simulink model "Sim3_Cart_OA"  (R2021b)
settings: Solver=VariableStepAuto  StartTime=0.0  StopTime=Inf  RelTol=1e-3
InitFcn:
  | run('settingParams.m')
undefined symbols (not defined in the file or in its folder): dt, Init_Direction, StartPoint, TurnPoint, Twist
libraries: robotlib x5, instrumentseriallib x4, simulink x1, realtime_pacer_lib x1
settings Model: Creator=shdet  LastModifiedBy=Hibik
settings SolverCC: AlgebraicLoopSolver=TrustRegion
settings DataIOCC: SaveOutput=off  SignalLogging=off  DSMLogging=off  SaveTime=off  ReturnWorkspaceOutputs=off
settings DebuggingCC: PregeneratedLibrarySubsystemCodeDiagnostic=none  SFMachineParentedDataDiag=warning  ArithmeticOperatorsInVariantConditions=warning
settings SFSimCC: SimUseLocalCustomCode=off  CustomCodeUndefinedFunction=UseInterfaceOnly
settings RTWCC: RTWUseLocalCustomCode=off

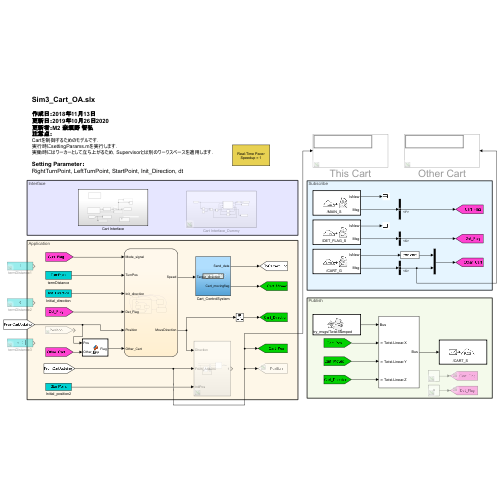
[thumbnail: Simulink's stored preview of the top-level diagram]
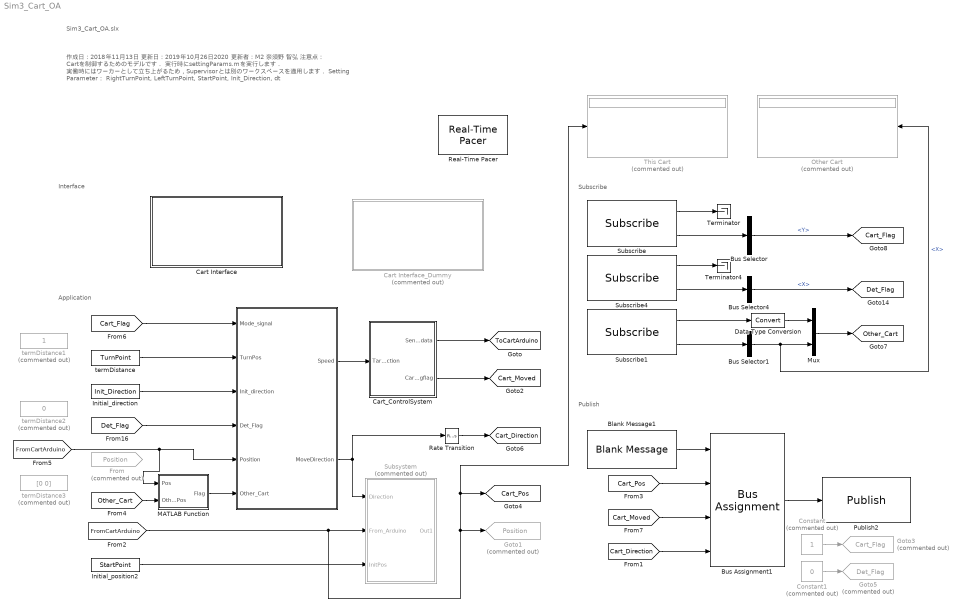
== system Sim3_Cart_OA ==
  note: 作成日：2018年11月13日
      | 更新日：2019年10月26日2020
      | 更新者：M2 奈須野 智弘
      | 注意点：
      | Cartを制御するためのモデルです．
      | 実行時にsettingParams.mを実行します．
      | 実働時にはワーカーとして立ち上がるため，Supervisorとは別のワークスペースを適用します．
      |
      | Setting Parameter：
      | RightTurnPoint, LeftTurnPoint, StartPoint, Init_Direction, dt
  note: Sim3_Cart_OA.slx
  note: Subscribe
  note: Publish
  note: Application
  note: Interface
  " " : Stateflow chart  TreatAsAtomicUnit=on
  Blank Message1 : robotlib/Blank Message  messageClass=Message  entityType=geometry_msgs/TwistStamped  messageType=geometry_msgs/TwistStamped  SampleTime=inf  legacyBusStruct=off
  Bus Assignment1 : BusAssignment  AssignedSignals=Twist.Linear.X,Twist.Linear.Y,Twist.Linear.Z
  Bus Selector : BusSelector  OutputSignals=Twist.Linear.Y
  Bus Selector1 : BusSelector  OutputSignals=Twist.Linear.X
  Bus Selector4 : BusSelector  OutputSignals=Twist.Linear.X
  Cart Interface : Subsystem
  Cart Interface_Dummy : Subsystem  Commented=on
  Cart_ControlSystem : Subsystem
  Constant : Constant  Commented=on  SampleTime=dt
  Constant1 : Constant  Commented=on  Value=0  SampleTime=dt
  Data Type Conversion : DataTypeConversion
  From : From  Commented=on  GotoTag=Position  TagVisibility=global
  Goto1 : Goto  Commented=on  GotoTag=Position  TagVisibility=global
  Goto3 : Goto  Commented=on  GotoTag=Cart_Flag  TagVisibility=global
  Goto5 : Goto  Commented=on  GotoTag=Det_Flag  TagVisibility=global
  Initial_direction : Constant  Value=Init_Direction  SampleTime=dt
  Initial_position2 : Constant  Value=StartPoint  SampleTime=dt
  MATLAB Function : MATLAB Function  TreatAsAtomicUnit=on
  Mux : Mux  Inputs=2
  Other Cart : Display  Commented=on
  Publish2 : robotlib/Publish  topicSource=Specify your own  topic=/CART_S  messageType=geometry_msgs/TwistStamped  legacyBusStruct=off  messageQueueLength=1
  Rate Transition : RateTransition
  Real-Time Pacer : realtime_pacer_lib/Real-Time Pacer  simTimePerRealTime=1
      settings: SourceProductName=Real-Time Pacer
  Subscribe : robotlib/Subscribe  topicSource=Specify your own  topic=/MAIN_S  messageType=geometry_msgs/TwistStamped  SampleTime=-1  legacyBusStruct=off  messageQueueLength=1
  Subscribe1 : robotlib/Subscribe  topicSource=Specify your own  topic=/CART_G  messageType=geometry_msgs/TwistStamped  SampleTime=-1  legacyBusStruct=off  messageQueueLength=1
  Subscribe4 : robotlib/Subscribe  topicSource=Specify your own  topic=/DET_FLAG_S  messageType=geometry_msgs/TwistStamped  SampleTime=-1  legacyBusStruct=off  messageQueueLength=1
  Subsystem : Subsystem  Commented=on
  Terminator : Terminator
  Terminator4 : Terminator
  This Cart : Display  Commented=on
  termDistance : Constant  Value=TurnPoint  SampleTime=dt
  termDistance1 : Constant  Commented=on  SampleTime=dt
  termDistance2 : Constant  Commented=on  Value=0  SampleTime=dt
  termDistance3 : Constant  Commented=on  Value=[0 0]  SampleTime=dt
  tag scope: Cart_Direction=global, Cart_Flag=global, Cart_Moved=global, Cart_Pos=global, Det_Flag=global, Other_Cart=global, ToCartArduino=global
  wires:
  Subscribe4/2 -> Bus Selector4/1
  Subscribe4/1 -> Terminator4/1
  [Cart_Pos] -> Bus Assignment1/2
  Bus Assignment1/1 -> Publish2/1
  Bus Selector4/1 -> [Det_Flag]  "<X>"
  Subscribe/1 -> Terminator/1
  [Cart_Moved] -> Bus Assignment1/3
  Blank Message1/1 -> Bus Assignment1/1
  Subscribe/2 -> Bus Selector/1
  Bus Selector/1 -> [Cart_Flag]  "<Y>"
  Cart_ControlSystem/2(Cart_movingflag) -> [Cart_Moved]
  Cart_ControlSystem/1(Send_data) -> [ToCartArduino]
  termDistance/1 -> " "/2(TurnPos)
  " "/1(Speed) -> Cart_ControlSystem/1(Target_direction)
  Initial_direction/1 -> " "/3(Init_direction)
  " "/2(MoveDirection) -> Rate Transition/1, Subsystem/1(Direction)
  [FromCartArduino] -> This Cart/1, [Cart_Pos], Goto1/1, Subsystem/2(From_Arduino)
  [Cart_Direction] -> Bus Assignment1/4
  Constant1/1 -> Goto5/1
  Constant/1 -> Goto3/1
  Bus Selector1/1 -> Other Cart/1, Mux/2  "<X>"
  Subscribe1/2 -> Bus Selector1/1
  Subscribe1/1 -> Data Type Conversion/1
  Mux/1 -> [Other_Cart]
  Data Type Conversion/1 -> Mux/1
  Rate Transition/1 -> [Cart_Direction]
  MATLAB Function/1(Flag) -> " "/6(Other_Cart)
  Initial_position2/1 -> Subsystem/3(InitPos)
  [FromCartArduino] -> MATLAB Function/1(Pos), " "/5(Position)
  [Cart_Flag] -> " "/1(Mode_signal)
  [Det_Flag] -> " "/4(Det_Flag)
  [Other_Cart] -> MATLAB Function/2(Other_Pos)

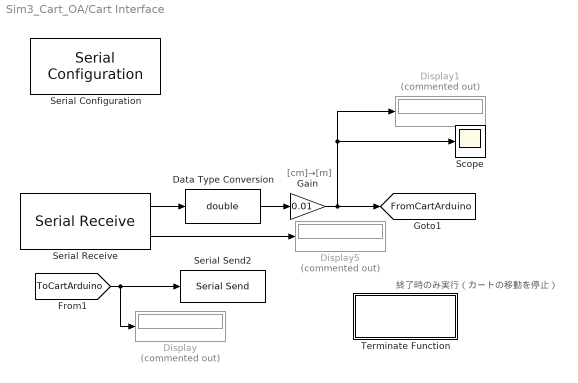
== system Sim3_Cart_OA/Cart Interface ==
  note: 終了時のみ実行（カートの移動を停止）
  note: [cm]→[m]
  Data Type Conversion : DataTypeConversion  OutDataTypeStr=double
  Display : Display  Commented=on
      settings: Format=binary (Stored Integer)
  Display1 : Display  Commented=on
  Display5 : Display  Commented=on
  Gain : Gain  Gain=0.01
  Scope : Scope
  Serial Configuration : instrumentseriallib/Serial Configuration  Priority=-200000  Port=COM5  ComPort=COM5  BaudRate=115200  DataBits=8  Parity=none  StopBits=1  ByteOrder=little-endian  FlowControl=none  Timeout=10  SimulateUsing=Interpreted execution  BlockInModel=on
  Serial Receive : instrumentseriallib/Serial Receive  Priority=1  Port=COM5  ComPort=COM5  DataType=int16  SaveDataType=uint8  ToggleHeader=off  Header=[]  ToggleTerminator=on  Terminator=<none>  CustomTerminator=[]  ToggleDataSize=on  DataSize=1  EnableBlockingMode=off  ActionDataUnavailable=Output last received value  ActionWhenDataUnavailable=Output last received value  CustomValue=-1  SampleTime=0.1  SimulateUsing=Interpreted execution  BlockInModel=on
  Serial Send2 : instrumentseriallib/Serial Send  Port=COM5  ComPort=COM5  Header=[]  Terminator=<none>  CustomTerminator=[]  EnableBlockingMode=off  SimulateUsing=Interpreted execution  BlockInModel=on
  Terminate Function : Subsystem  TreatAsAtomicUnit=on
  tag scope: FromCartArduino=global
  wires:
  [ToCartArduino] -> Serial Send2/1, Display/1
  Gain/1 -> Scope/1, Display1/1, [FromCartArduino]
  Serial Receive/1 -> Data Type Conversion/1
  Data Type Conversion/1 -> Gain/1
  Serial Receive/2 -> Display5/1

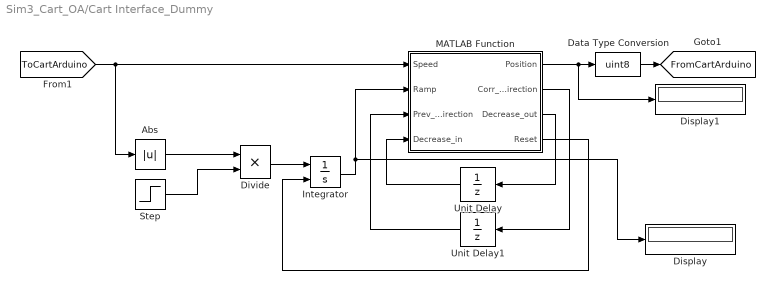
== system Sim3_Cart_OA/Cart Interface_Dummy ==
  Abs : Abs
  Data Type Conversion : DataTypeConversion  OutDataTypeStr=uint8
  Display : Display
  Display1 : Display
      settings: Format=binary (Stored Integer)
  Divide : Product  Inputs=**
  Integrator : Integrator  ExternalReset=rising
  MATLAB Function : MATLAB Function  TreatAsAtomicUnit=on
  Step : Step  Time=0  After=0.5  SampleTime=0
  Unit Delay : UnitDelay  SampleTime=-1  HasFrameUpgradeWarning=on
  Unit Delay1 : UnitDelay  SampleTime=-1  HasFrameUpgradeWarning=on
  tag scope: FromCartArduino=global
  wires:
  MATLAB Function/3(Decrease_out) -> Unit Delay/1
  MATLAB Function/2(Corr_Direction) -> Unit Delay1/1
  Unit Delay/1 -> MATLAB Function/4(Decrease_in)
  Unit Delay1/1 -> MATLAB Function/3(Prev_Direction)
  MATLAB Function/1(Position) -> Data Type Conversion/1, Display1/1
  [ToCartArduino] -> Abs/1, MATLAB Function/1(Speed)
  MATLAB Function/4(Reset) -> Integrator/2
  Step/1 -> Divide/2
  Data Type Conversion/1 -> [FromCartArduino]
  Divide/1 -> Integrator/1
  Abs/1 -> Divide/1
  Integrator/1 -> Display/1, MATLAB Function/2(Ramp)

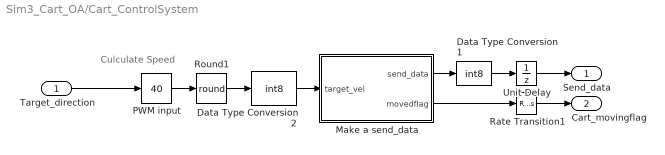
== system Sim3_Cart_OA/Cart_ControlSystem ==
  note: Culculate Speed
  Target_direction : Inport
  Data Type Conversion1 : DataTypeConversion  OutDataTypeStr=int8
  Data Type Conversion2 : DataTypeConversion  OutDataTypeStr=int8
  Make a send_data : MATLAB Function  TreatAsAtomicUnit=on
  PWM input : simulink/Math Operations/Slider Gain  gain=40  low=0  high=127
  Rate Transition1 : RateTransition
  Round1 : Rounding  Operator=round
  Unit Delay : UnitDelay  SampleTime=-1  HasFrameUpgradeWarning=on
  Send_data : Outport  VectorParamsAs1DForOutWhenUnconnected=off
  Cart_movingflag : Outport  Port=2  VectorParamsAs1DForOutWhenUnconnected=off
  wires:
  PWM input/1 -> Round1/1
  Make a send_data/2(movedflag) -> Rate Transition1/1
  Data Type Conversion2/1 -> Make a send_data/1(target_vel)
  Data Type Conversion1/1 -> Unit Delay/1
  Target_direction/1 -> PWM input/1
  Round1/1 -> Data Type Conversion2/1
  Make a send_data/1(send_data) -> Data Type Conversion1/1
  Unit Delay/1 -> Send_data/1
  Rate Transition1/1 -> Cart_movingflag/1

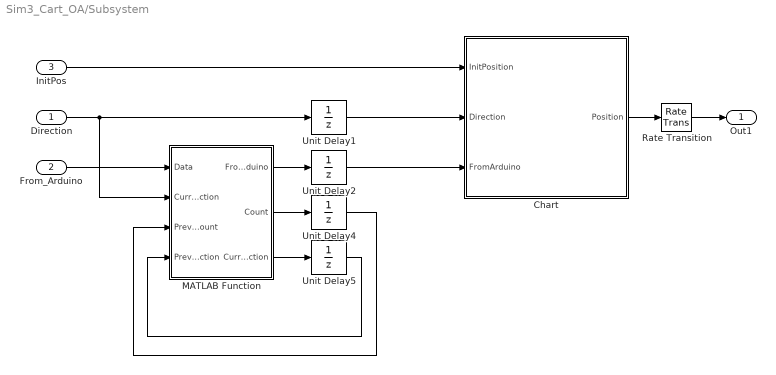
== system Sim3_Cart_OA/Subsystem ==
  Direction : Inport
  From_Arduino : Inport  Port=2
  InitPos : Inport  Port=3
  Chart : Stateflow chart  TreatAsAtomicUnit=on
  MATLAB Function : MATLAB Function  TreatAsAtomicUnit=on
  Rate Transition : RateTransition
  Unit Delay{1..2,4..5} (4 alike) : UnitDelay  SampleTime=-1  HasFrameUpgradeWarning=on
  Out1 : Outport  VectorParamsAs1DForOutWhenUnconnected=off
  wires:
  From_Arduino/1 -> MATLAB Function/1(Data)
  MATLAB Function/2(Count) -> Unit Delay4/1
  MATLAB Function/3(Curr_Direction) -> Unit Delay5/1
  Unit Delay5/1 -> MATLAB Function/4(Prev_Direction)
  Unit Delay4/1 -> MATLAB Function/3(Prev_Count)
  Direction/1 -> Unit Delay1/1, MATLAB Function/2("Curr_Direction ")
  MATLAB Function/1(FromArduino) -> Unit Delay2/1
  Chart/1(Position) -> Rate Transition/1
  InitPos/1 -> Chart/1(InitPosition)
  Unit Delay1/1 -> Chart/2(Direction)
  Unit Delay2/1 -> Chart/3(FromArduino)
  Rate Transition/1 -> Out1/1

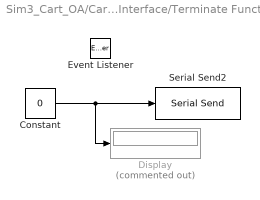
== system Sim3_Cart_OA/Cart Interface/Terminate Function ==
  Constant : Constant  Value=0  OutDataTypeStr=uint8
  Display : Display  Commented=on
      settings: Format=binary (Stored Integer)
  Event Listener : EventListener  DisableCoverage=on  EventType=Terminate  EventName=reset
  Serial Send2 : instrumentseriallib/Serial Send  Port=COM5  ComPort=COM5  Header=[]  Terminator=<none>  CustomTerminator=[]  EnableBlockingMode=off  SimulateUsing=Interpreted execution  BlockInModel=on
  wires:
  Constant/1 -> Serial Send2/1, Display/1

== matlab function Sim3_Cart_OA/MATLAB Function ==
  data: Pos input; Flag output; Other_Pos input
function Flag = fcn(Pos, Other_Pos)

if Other_Pos(1) == 0
    Flag = 0;
else
    if abs(Other_Pos(2) - Pos) < 0.95 && Pos > 0.0
        Flag = 1;
    else
        Flag = 0;
    end
end

== matlab function Sim3_Cart_OA/Cart Interface_Dummy/MATLAB Function ==
  data: Speed input; Position output; Corr_Direction output; Ramp input; Prev_Direction input; Decrease_in input; Decrease_out output; Reset output
function [Position, Corr_Direction,Decrease_out, Reset] = fcn(Speed,Ramp,Prev_Direction,Decrease_in)
flag = 0;

if Speed > 0
    Corr_Direction = 1;
elseif Speed < 0
    Corr_Direction = -1;
else
    Corr_Direction = Prev_Direction;
end

if Ramp < Decrease_in
    Decrease_out = 0;
else
    Decrease_out = Decrease_in;
end

Posit = uint8(Ramp - Decrease_out);

if Corr_Direction * Prev_Direction == 1
    flag = 0;
    Reset = 0;
    if Posit >= 100
        flag = 1;
        Decrease_out = Decrease_in + 100;
        Posit = uint8(Ramp - Decrease_out);
    end
else
    Reset = 1;
    Posit = uint8(0);
end

Position = uint8(bitshift(flag,7)+Posit);

== stateflow chart Sim3_Cart_OA/Subsystem/Chart ==
  state Stop/
    entry:
    Position = Position;
  state WaitTime1/
    entry:
    Position = Position;
  state Move_Left/
    entry:
    Prev_Direction = 1;
    Position = TurnPos - ((FromArduino(1) * 100) + FromArduino(2)) / 100;
  state Move_Right/
    entry:
    Prev_Direction = -1;
    Position = TurnPos + (FromArduino(1) * 100 + FromArduino(2)) / 100;
  state WaitTime2/
    entry:
    Position = Position;
  (default) -> Stop : {
      | Position = InitPosition;
      | TurnPos = InitPosition;
      | }
  Stop -> Move_Left [order 1] : [Direction == 1]
  Move_Right -> Stop [order 2] : [Direction == 0]
  Stop -> Move_Right [order 2] : [Direction == -1]
  Move_Left -> Stop [order 2] : [Direction == 0]
  Move_Right -> WaitTime1 [order 1] : [Direction == 1]
      | {TurnPos = Position;}
  WaitTime1 -> Move_Left : after(1.5,sec)
  Move_Left -> Move_Left [order 3] : [Direction == 1]
  Move_Right -> Move_Right [order 3] : [Direction == -1]
  WaitTime2 -> Move_Right : after(1.5,sec)
  Move_Left -> WaitTime2 [order 1] : [Direction == -1]
      | {TurnPos = Position;}
  data: InitPosition input; Direction input; FromArduino input; Position output; Prev_Direction local double; TurnPos local

== matlab function Sim3_Cart_OA/Subsystem/MATLAB Function ==
  data: Data input; FromArduino output; Curr_Direction input; Prev_Count input; Prev_Direction input; Count output; Curr_Direction output
function [FromArduino, Count, Curr_Direction] = fcn(Data, Curr_Direction, Prev_Count, Prev_Direction)
% 入力(data)を右に7bitシフトして、上位1bitを取り出す
Flag = double(bitshift(Data,-7));

% 入力(data)と127(01111111)のAND演算をして、下位7bitを取り出す
Distance = double(bitand(Data, 127));

% Check Parameters
if Curr_Direction * Prev_Direction == -1
    Count = 0;
elseif Flag == 1
    Count = Prev_Count + 1;
else
    Count = Prev_Count;
end

FromArduino = [Count, Distance];

== stateflow chart Sim3_Cart_OA/  ==
  state Wait/
    entry:Speed=0;
  state Movable/
    entry:
    state check/
    state Right/
      entry:
      Speed = -1;
      MoveDirection = -1;
    state Left/
      entry:
      Speed = 1;
      MoveDirection = 1;
    state ChangeDirection/
      entry:
      MoveDirection = -1 * MoveDirection;
    (default) -> check
    check -> Left [order 1] : [MoveDirection == 1]
    check -> Right [order 2] : [MoveDirection == -1]
    Right -> ChangeDirection : [Position >= TurnPos(1)-0.1]
    Left -> ChangeDirection : [Position <= TurnPos(2)+0.1]
  state OtherCart_Near/
    entry:
    Speed = 0;
  state OtherCart_Near1/
    entry:
    MoveDirection = -1 * MoveDirection;
    Speed = MoveDirection;
  (default) -> Wait : {
      | Speed = 0;
      | MoveDirection=Init_direction;
      | }
  OtherCart_Near1 -> Wait [order 2] : [Mode_signal == 0 || Det_Flag == 1]
  OtherCart_Near -> Wait [order 2] : [Mode_signal == 0 || Det_Flag == 1]
  Movable -> Wait [order 1] : [Mode_signal == 0 || Det_Flag == 1]
  ChangeDirection -> Wait
  Wait -> Movable : after(1.0,sec)
      | [Mode_signal == 1 && Det_Flag ~= 1 && Other_Cart == 0]
  Movable -> OtherCart_Near [order 2] : [Other_Cart == 1]
  OtherCart_Near -> OtherCart_Near1 [order 1] : after(5.0,sec)
  OtherCart_Near1 -> Movable [order 1] : [Other_Cart == 0]
  data: Mode_signal input; Speed output; TurnPos input; MoveDirection output; Init_direction input; Det_Flag input; Position input; Other_Cart input

== matlab function Sim3_Cart_OA/Cart_ControlSystem/Make a send_data ==
  data: send_data output; target_vel input; movedflag output
function [send_data,movedflag] = fcn(target_vel)

send_data = target_vel;

if(target_vel == 0)
    movedflag = 1;
else
    movedflag = 0;
end
